simulink model "lugre"  (R2019b)
settings: Solver=ode15s  StartTime=0.0  StopTime=30  MaxStep=1e-3  RelTol=1e-3
values from neighbouring files (symbols this model uses):
  Fc_stim = Fc*0.99    (= 0.594)    [motor_data.m]
  st = 1e-3    (= 0.001)    [motor_data.m]    (also in tuning_pi.m = 0.000125)
libraries: fl_lib x5, nesl_utility x4, simulink x1
settings Model: Creator=manue  LastModifiedBy=manue

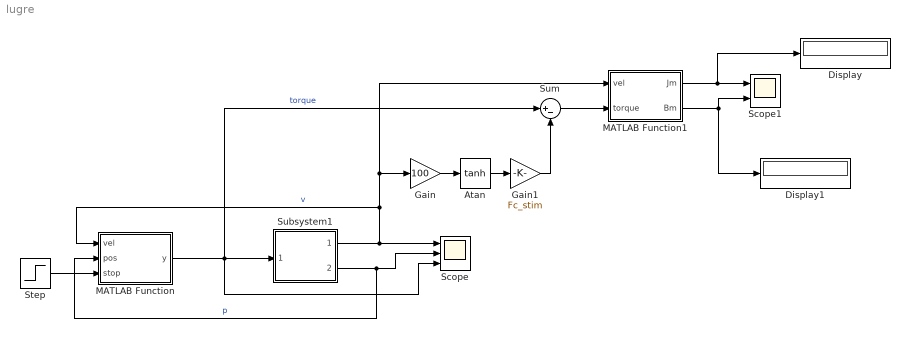
== system lugre ==
  Atan : Trigonometry  Operator=tanh
  Display : Display
  Display1 : Display
  Gain : Gain  Gain=100
  Gain1 : Gain  Gain=Fc_stim
  MATLAB Function : MATLAB Function  TreatAsAtomicUnit=on  SystemSampleTime=1e-3
  MATLAB Function1 : MATLAB Function  TreatAsAtomicUnit=on  SystemSampleTime=1e-3
  Scope : Scope  NumInputPorts=3
  Scope1 : Scope  NumInputPorts=2
  Step : Step  Time=20  SampleTime=0
  Subsystem1 : Subsystem
  Sum : Sum  Inputs=|+-
  wires:
  MATLAB Function/1(y) -> Sum/1, Scope/3, Subsystem1/1(torque)  "torque"
  Subsystem1/1(velocity) -> Gain/1, MATLAB Function1/1(vel), MATLAB Function/1(vel), Scope/1  "v"
  Subsystem1/2("position ") -> MATLAB Function/2(pos), Scope/2  "p"
  MATLAB Function1/1(Jm) -> Display/1, Scope1/1
  MATLAB Function1/2(Bm) -> Display1/1, Scope1/2
  Sum/1 -> MATLAB Function1/2(torque)
  Gain/1 -> Atan/1
  Atan/1 -> Gain1/1
  Gain1/1 -> Sum/2
  Step/1 -> MATLAB Function/3(stop)

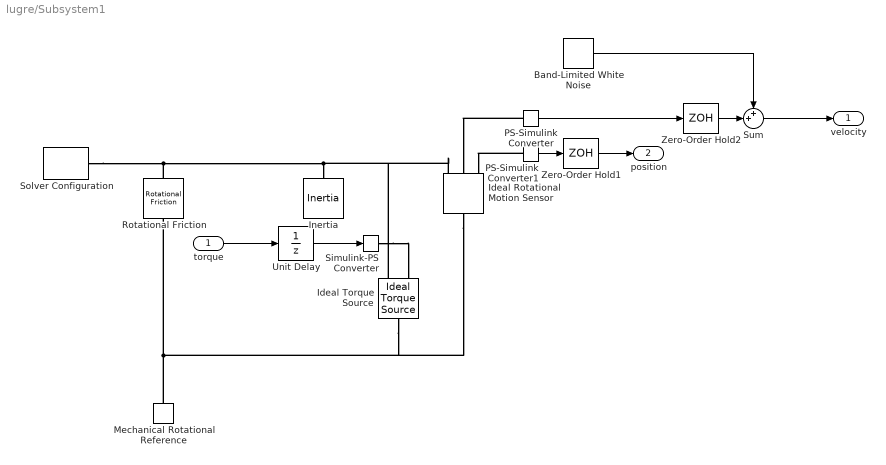
== system lugre/Subsystem1 ==
  torque : Inport
  Band-Limited White Noise : simulink/Sources/Band-Limited White Noise  Cov=noise  Ts=st  seed=[23341]
  Ideal Rotational Motion Sensor : fl_lib/Mechanical/Mechanical Sensors/Ideal Rotational Motion Sensor  offset=0 rad
  Ideal Torque Source : fl_lib/Mechanical/Mechanical Sources/Ideal Torque Source
  Inertia : fl_lib/Mechanical/Rotational Elements/Inertia  inertia=J kg*m^2  w_specify=off  w_priority=High  w=0 rad/s  w_nominal_specify=off  w_nominal_unit=rad/s  w_nominal_value=1  t_specify=off  t_priority=None  t=0 N*m  t_nominal_specify=off  t_nominal_unit=N*m  t_nominal_value=1
  Mechanical Rotational Reference : fl_lib/Mechanical/Rotational Elements/Mechanical Rotational Reference
  PS-Simulink Converter : nesl_utility/PS-Simulink Converter  PhysicalDomain=network_engine_domain  SubClassName=ps_output  LeftPortType=input  RightPortType=output  PseudoPeriodic=off  Frequencies=[]  Unit=rad/s  AffineConversion=off
  PS-Simulink Converter1 : nesl_utility/PS-Simulink Converter  PhysicalDomain=network_engine_domain  SubClassName=ps_output  LeftPortType=input  RightPortType=output  PseudoPeriodic=off  Frequencies=[]  Unit=rad  AffineConversion=off
  Rotational Friction : fl_lib/Mechanical/Rotational Elements/Rotational Friction  brkwy_trq=Fs N*m  brkwy_vel=vs rad/s  Col_trq=Fc N*m  visc_coef=Bm N*m/(rad/s)  w_specify=off  w_priority=None  w=0 rad/s  w_nominal_specify=off  w_nominal_unit=rad/s  w_nominal_value=1  t_specify=off  t_priority=None  t=0 N*m  t_nominal_specify=off  t_nominal_unit=N*m  t_nominal_value=1
      settings: SourceProductName=Simscape
  Simulink-PS Converter : nesl_utility/Simulink-PS Converter  PhysicalDomain=network_engine_domain  SubClassName=ps_input  LeftPortType=input  RightPortType=output  PseudoPeriodic=off  Frequencies=[]  NoiseDistribution=none  NoiseParameters=[]  Unit=N*m  AffineConversion=off  FilteringAndDerivatives=provide  SimscapeFilterOrder=1  InputFilterTimeConstant=0.001  UdotUserProvided=0
  Solver Configuration : nesl_utility/Solver Configuration  PhysicalDomain=network_engine_domain  SubClassName=solver  LeftPortType=input  RightPortType=generic  Tones=[]  Harmonics=[]  SimulateNoise=off  Profile=off  UseLocalSampling=off  EnableSwitchedLinearOptims=on  FrequencyDomain=off  UseCCode=off  RelTol=0.001  AbsTol=1e-06  MinStep=1e-09  ToWorkspace=off  RevertToSquareIcSolve=off  NumHomotopyIterations=100  PhasorMode=off  PhasorModeNumHarmonics=1  DoDC=off  ResidualTolerance=1e-09  UseLocalSolver=off  LocalSolverChoice=NE_BACKWARD_EULER_ADVANCER  LocalSolverSampleTime=0.001  DoFixedCost=off  MaxNonlinIter=3  MaxModeIter=2  LinearAlgebra=auto  EquationFormulation=NE_TIME_EF  DelaysMemoryBudget=1024  AutomaticFiltering=on  FilteringTimeConstant=0.001  PartitionStorageMethod=AS_NEEDED  PartitionMemoryBudget=1024  PartitionMethod=ROBUST
  Sum : Sum  Inputs=++|
  Unit Delay : UnitDelay  SampleTime=st  HasFrameUpgradeWarning=on
  Zero-Order Hold1 : ZeroOrderHold  SampleTime=st
  Zero-Order Hold2 : ZeroOrderHold  SampleTime=st
  velocity : Outport
  "position " : Outport  Port=2
  wires:
  PS-Simulink Converter/1 -> Zero-Order Hold2/1
  PS-Simulink Converter1/1 -> Zero-Order Hold1/1
  torque/1 -> Unit Delay/1
  Unit Delay/1 -> Simulink-PS Converter/1
  Zero-Order Hold1/1 -> "position "/1
  Zero-Order Hold2/1 -> Sum/2
  Sum/1 -> velocity/1
  Band-Limited White Noise/1 -> Sum/1
  connections:
  Rotational Friction/RConn1 -- Ideal Torque Source/RConn2 -- Ideal Rotational Motion Sensor/RConn1 -- Inertia/LConn1 -- Solver Configuration/RConn1
  Mechanical Rotational Reference/LConn1 -- Ideal Torque Source/LConn1 -- Ideal Rotational Motion Sensor/LConn1 -- Rotational Friction/LConn1
  Simulink-PS Converter/RConn1 -- Ideal Torque Source/RConn1
  PS-Simulink Converter/LConn1 -- Ideal Rotational Motion Sensor/RConn2
  PS-Simulink Converter1/LConn1 -- Ideal Rotational Motion Sensor/RConn3

== matlab function lugre/MATLAB Function1 ==
  data: vel input; Jm output; torque input; Bm output
function [Jm,Bm] = rls(vel,torque)
Jm=0;
Bm=0;
filt=0.9;
persistent Q S st param vel_filt torque_filt;
if isempty(Q)
    Q=eye(2);
    S=30;
    st=1e-3;
    param=[0;0];
    vel_filt=vel;
    torque_filt=torque;
end

%acc=(vel-vel_prec)/st;
vel_filt_new=filt*vel_filt+(1-filt)*vel;
acc=(vel_filt_new-vel_filt)/st;
torque_filt=filt*torque_filt+(1-filt)*torque;

Q(1,1)=Q(1,1)+S*acc^2;
Q(1,2)=Q(1,2)+S*acc*vel_filt_new;
Q(2,1)=Q(1,2);
Q(2,2)=Q(2,2)+S*vel_filt_new^2;

innovation=torque_filt-(param(1)*acc+param(2)*vel);

param(1)=param(1)+ (S*(acc*Q(2,2) - Q(1,2)*vel_filt_new))/(- Q(1,2)^2 + Q(1,1)*Q(2,2))  * innovation;
param(2)=param(2)- (S*(acc*Q(1,2) - Q(1,1)*vel_filt_new))/(- Q(1,2)^2 + Q(1,1)*Q(2,2))  * innovation;

Jm=param(1);
Bm=param(2);
vel_filt=vel_filt_new;

== matlab function lugre/MATLAB Function ==
  data: vel input; pos input; y output; stop input
function y = fcn(vel,pos,stop)
y=0;

vel_max=50;
vel_min=-vel_max;
pos_max=1;
pos_min=-5;
hist=0.1;
max_torque=12;
static_friction=0.6;

pos_mean=0.5*(pos_max+pos_min);
hysteresis=(pos_max-pos_mean)*hist;
pos_threshold=pos_mean+hysteresis;
neg_threshold=pos_mean-hysteresis;


vel_percentage=0.5;

persistent state torque stopping;
if isempty(state)
    
    state=-1;
    torque=0;
    stopping=0;
end


if (stop && not(stopping))
    stopping=1;
    if (vel>0)
        state=99;
        torque=-max_torque;
    else
        state=98;
        torque=max_torque;
    end
elseif (state==-1)
    if (pos>pos_mean)
        state=0;
        torque=-(static_friction+(max_torque-static_friction)*0.2);
    else
        state=1;
        torque=static_friction+(max_torque-static_friction)*0.2;
    end
elseif (state==99 && vel<0)
    state=100;
    torque=0;
elseif (state==98 && vel>0)
    state=100;
    torque=0;
elseif (state==0 && pos<pos_mean)
    state=3;
elseif (state==1 && pos>pos_mean)
    state=2;
elseif ((state==2 && pos>pos_threshold) || vel>vel_max*vel_percentage)
    torque=-max_torque;
    state=4;
elseif ((state==3 && pos<neg_threshold) || vel<vel_min*vel_percentage)
    torque=max_torque;
    state=5;
elseif ((state==4) && vel<0)
    torque=-(static_friction+(max_torque-static_friction)*(0.2+0.5*rand));
    state=3;
elseif ((state==5) && vel>0)
    torque=(static_friction+(max_torque-static_friction)*(0.2+0.5*rand));
    state=2;
end
y=torque;
